simulink model "mmawe"  (Simulink 3.00)
settings: Solver=ode45  SolverMode=SingleTasking  StartTime=0.0  StopTime=20  MaxStep=0.01  RelTol=0.1  AbsTol=1e-2
values from neighbouring files (symbols this model uses):
  dci = [2 8 16 16]    [awu.mat]    (also in awup.m = dcy/dcy(1))
  nc11ii = [5 10 8]    [awu.mat]
  nc12ii = [-5 -15 -16]    [awu.mat]
  nc21ii = [-3 -3 0]    [awu.mat]
  nc22ii = [5 10 8]    [awu.mat]
  ns1 = 2.5    [awu.mat]
  tau = 0.1    [awu.mat]
settings Model: TimeSaveName=t  SaveOutput=off

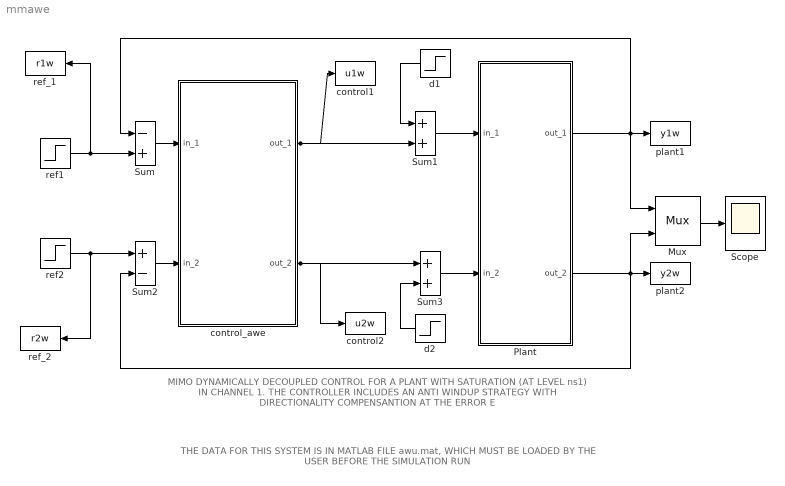
== system mmawe ==
  note: MIMO DYNAMICALLY DECOUPLED CONTROL
      |  FOR A PLANT WITH SATURATION  (AT LEVEL ns1) IN CHANNEL 1.
      | THE CONTROLLER INCLUDES AN ANTI WINDUP STRATEGY
      | WITH  DIRECTIONALITY COMPENSANTION  AT  THE  ERROR  E
  note: THE DATA FOR THIS SYSTEM IS IN MATLAB FILE awu.mat,
      | WHICH MUST BE LOADED BY THE USER BEFORE THE SIMULATION RUN
  Mux : Mux  Inputs=2
      settings: DisplayOption=none
  Plant : Subsystem
      mask Type: PLANT
      mask Display: disp('PLANT')
  Scope : Scope
      settings: TickLabels=on  TimeRange=20.000000  YMin=-3.000000  YMax=3.000000  SaveToWorkspace=off  SaveName=ScopeData  DataFormat=Matrix
  Sum : Sum  Inputs=-+  SaturateOnIntegerOverflow=on
  Sum1 : Sum  Inputs=++  SaturateOnIntegerOverflow=on
  Sum2 : Sum  Inputs=+-  SaturateOnIntegerOverflow=on
  Sum3 : Sum  Inputs=++  SaturateOnIntegerOverflow=on
  control1 : ToWorkspace  VariableName=u1w  SampleTime=0  SaveFormat=Matrix
      settings: Buffer=10000
  control2 : ToWorkspace  VariableName=u2w  SampleTime=0  SaveFormat=Matrix
      settings: Buffer=10000
  control_awe : Subsystem
      mask Type: Control
      mask Display: disp('Control AWE')
  d1 : Step  Orientation=left  Time=5  Before=0  After=0  SampleTime=0
  d2 : Step  Orientation=left  Time=15  Before=0  After=0  SampleTime=0
  plant1 : ToWorkspace  VariableName=y1w  SampleTime=0  SaveFormat=Matrix
      settings: Buffer=10000
  plant2 : ToWorkspace  VariableName=y2w  SampleTime=0  SaveFormat=Matrix
      settings: Buffer=10000
  ref1 : Step  Time=1  Before=0  After=1  SampleTime=0
  ref2 : Step  Time=10  Before=0  After=1.5  SampleTime=0
  ref_1 : ToWorkspace  VariableName=r1w  SampleTime=0  SaveFormat=Matrix
      settings: Buffer=10000
  ref_2 : ToWorkspace  VariableName=r2w  SampleTime=0  SaveFormat=Matrix
      settings: Buffer=10000
  wires:
  Sum/1 -> control_awe/1(in_1)
  Mux/1 -> Scope/1
  Sum1/1 -> Plant/1(in_1)
  Sum3/1 -> Plant/2(in_2)
  d1/1 -> Sum1/1
  Sum2/1 -> control_awe/2(in_2)
  ref1/1 -> Sum/2, ref_1/1
  Plant/1(out_1) -> plant1/1, Mux/1, Sum/1
  Plant/2(out_2) -> plant2/1, Mux/2, Sum2/2
  ref2/1 -> Sum2/1, ref_2/1
  control_awe/1(out_1) -> Sum1/2, control1/1
  control_awe/2(out_2) -> Sum3/1, control2/1
  d2/1 -> Sum3/2

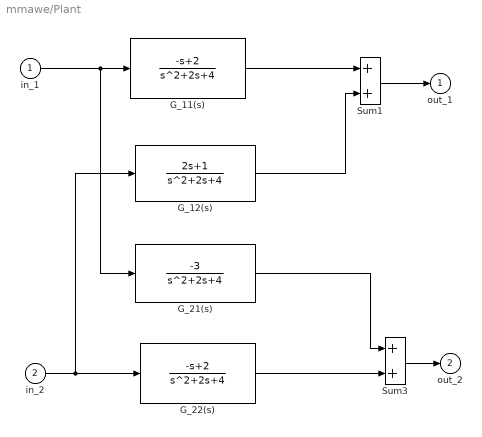
== system mmawe/Plant ==
  in_1 : Inport  Port=1  PortWidth=-1  SampleTime=-1  DataType=auto
      settings: SignalType=auto
  in_2 : Inport  Port=2  PortWidth=-1  SampleTime=-1  DataType=auto
      settings: SignalType=auto
  G_11(s) : TransferFcn  Numerator=[-1 2]  Denominator=[1 2 4]
  G_12(s) : TransferFcn  Numerator=[2 1]  Denominator=[1 2 4]
  G_21(s) : TransferFcn  Numerator=-3  Denominator="[1 2  4]"
  G_22(s) : TransferFcn  Numerator="[-1  2]"  Denominator="[1  2   4]"
  Sum1 : Sum  Inputs=++  SaturateOnIntegerOverflow=on
  Sum3 : Sum  Inputs=++  SaturateOnIntegerOverflow=on
  out_1 : Outport  Port=1  InitialOutput=0
  out_2 : Outport  Port=2  InitialOutput=0
  wires:
  G_12(s)/1 -> Sum1/2
  G_11(s)/1 -> Sum1/1
  G_21(s)/1 -> Sum3/1
  G_22(s)/1 -> Sum3/2
  in_1/1 -> G_11(s)/1, G_21(s)/1
  in_2/1 -> G_22(s)/1, G_12(s)/1
  Sum1/1 -> out_1/1
  Sum3/1 -> out_2/1

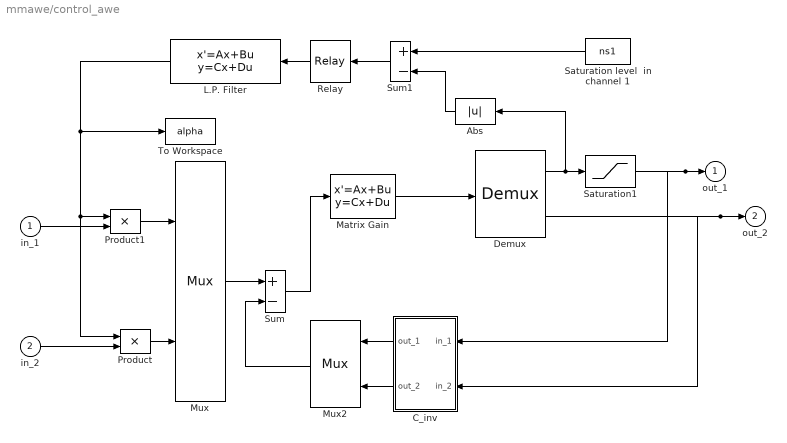
== system mmawe/control_awe ==
  in_1 : Inport  Port=1  PortWidth=-1  SampleTime=-1  DataType=auto
      settings: SignalType=auto
  in_2 : Inport  Port=2  PortWidth=-1  SampleTime=-1  DataType=auto
      settings: SignalType=auto
  Abs : Abs  Orientation=left
  C_inv : Subsystem  Orientation=left
      mask Type: C_inv
      mask Display: disp('C_inv')
  Demux : Demux  Outputs=2
  "L.P. Filter  " : StateSpace  Orientation=left  A=-1/tau  B=1/tau  C=1  D=0  X0=1
  Matrix Gain : StateSpace  A=[]  B=[]  C=[]  D=K  X0=0  mask(Matrix Gain){@1=cinf}
      mask prompts: @1 "Gain matrix:"
      mask help: Matrix Gain.
      mask init:
      | K = @1;
      mask Help: Multiplies input vector by entered matrix to produce output vector (y=Au).
      mask Display: disp('c_inf')
  Mux : Mux  Inputs=2
      settings: DisplayOption=none
  Mux2 : Mux  Orientation=left  Inputs=2
      settings: DisplayOption=none
  Product : Product  Inputs=2  SaturateOnIntegerOverflow=on
  Product1 : Product  Inputs=2  SaturateOnIntegerOverflow=on
  Relay : Relay  Orientation=left  OnSwitchValue=0.01  OffSwitchValue=-0.01  OnOutputValue=1  OffOutputValue=0
  Saturation level  in channel 1 : Constant  Orientation=left  Value=ns1
  Saturation1 : Saturate  UpperLimit=ns1  LowerLimit=-ns1
  Sum : Sum  Inputs=+-  SaturateOnIntegerOverflow=on
  Sum1 : Sum  Orientation=left  Inputs=+-  SaturateOnIntegerOverflow=on
  To Workspace : ToWorkspace  VariableName=alpha  SampleTime=0  SaveFormat=Matrix
      settings: Buffer=10000
  out_1 : Outport  Port=1  InitialOutput=0
  out_2 : Outport  Port=2  InitialOutput=0
  wires:
  Matrix Gain/1 -> Demux/1
  Mux/1 -> Sum/1
  C_inv/1(out_1) -> Mux2/1
  C_inv/2(out_2) -> Mux2/2
  Product1/1 -> Mux/1
  in_1/1 -> Product1/2
  Product/1 -> Mux/2
  in_2/1 -> Product/2
  Relay/1 -> "L.P. Filter  "/1
  Sum1/1 -> Relay/1
  Saturation level  in channel 1/1 -> Sum1/1
  Abs/1 -> Sum1/2
  Mux2/1 -> Sum/2
  Sum/1 -> Matrix Gain/1
  Demux/2 -> out_2/1, C_inv/2(in_2)
  Saturation1/1 -> out_1/1, C_inv/1(in_1)
  "L.P. Filter  "/1 -> Product/1, Product1/1, To Workspace/1
  Demux/1 -> Saturation1/1, Abs/1

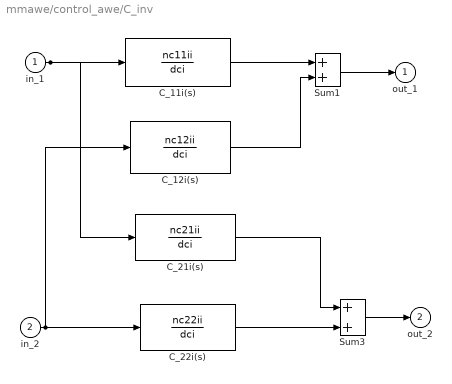
== system mmawe/control_awe/C_inv ==
  in_1 : Inport  Port=1  PortWidth=-1  SampleTime=-1  DataType=auto
      settings: SignalType=auto
  in_2 : Inport  Port=2  PortWidth=-1  SampleTime=-1  DataType=auto
      settings: SignalType=auto
  C_11i(s) : TransferFcn  Numerator=nc11ii  Denominator=dci
  C_12i(s) : TransferFcn  Numerator=nc12ii  Denominator=dci
  C_21i(s) : TransferFcn  Numerator=nc21ii  Denominator=dci
  C_22i(s) : TransferFcn  Numerator=nc22ii  Denominator=dci
  Sum1 : Sum  Inputs=++  SaturateOnIntegerOverflow=on
  Sum3 : Sum  Inputs=++  SaturateOnIntegerOverflow=on
  out_1 : Outport  Port=1  InitialOutput=0
  out_2 : Outport  Port=2  InitialOutput=0
  wires:
  in_2/1 -> C_12i(s)/1, C_22i(s)/1
  C_22i(s)/1 -> Sum3/2
  C_21i(s)/1 -> Sum3/1
  C_11i(s)/1 -> Sum1/1
  C_12i(s)/1 -> Sum1/2
  Sum1/1 -> out_1/1
  in_1/1 -> C_11i(s)/1, C_21i(s)/1
  Sum3/1 -> out_2/1
